simulink model "gm_sampleModel1484_1_sub_sub"  (R2023a)
settings: Solver=VariableStepAuto  StartTime=0.0  StopTime=10.0  RelTol=1e-3
libraries: hdlsllib x8, simulink x2
settings Model: Creator=user1  LastModifiedBy=user1
settings OptimizationCC: BlockReduction=off  ConditionallyExecuteInputs=off
settings DebuggingCC: InheritedTsInSrcMsg=none

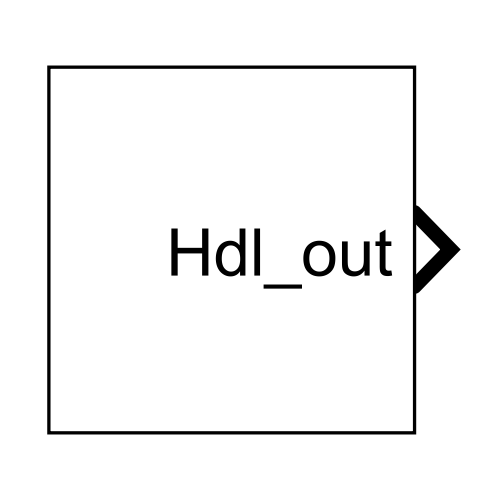
[thumbnail: Simulink's stored preview of the top-level diagram]
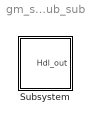
== system gm_sampleModel1484_1_sub_sub ==
  Subsystem : Subsystem

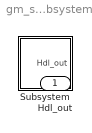
== system gm_sampleModel1484_1_sub_sub/Subsystem ==
  Subsystem : Subsystem
  Hdl_out : Outport  OutDataTypeStr=uint8

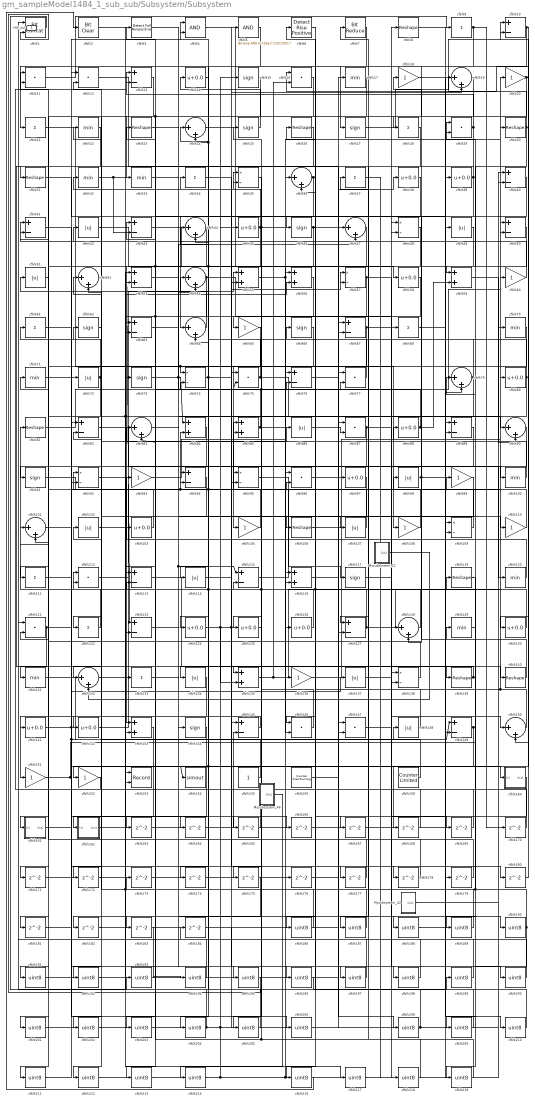
== system gm_sampleModel1484_1_sub_sub/Subsystem/Subsystem ==
  Mysubsystem_22 : Subsystem  TreatAsAtomicUnit=on  RTWFcnName=Mysubsystem_22
      settings: RTWFcnNameOpts=User specified  RTWFileNameOpts=Use function name
  Mysubsystem_42 : Subsystem  TreatAsAtomicUnit=on  RTWFcnName=Mysubsystem_42
      settings: RTWFcnNameOpts=User specified  RTWFileNameOpts=Use function name
  Mysubsystem_46 : Subsystem  TreatAsAtomicUnit=on  RTWFcnName=Mysubsystem_46
      settings: RTWFcnNameOpts=User specified  RTWFileNameOpts=Use function name
  cfblk1 : hdlsllib/Logic and Bit Operations/Bit Concat  numInputs=2
  cfblk{10,13,40..41,43,50,63,67,76,82,89,94,113,115,123,127,145,149} (18 alike) : Sum  Inputs=+-  OutDataTypeStr=uint8
  cfblk{17,22,32..33,70..71,100,120,129,131} (10 alike) : MinMax  OutDataTypeStr=uint8
  cfblk{19,24,36,44,47,52,54,64,79,83,90,101,128,132,150} (15 alike) : Sum  Inputs=|++  OutDataTypeStr=uint8
  cfblk{42,49,51,72,86,98,102,107,114,134,137,148} (12 alike) : Abs  OutDataTypeStr=uint8  SaturateOnIntegerOverflow=off
  cfblk{14,38..39,45,58,80,88,97,103,124..126,130,141..142} (15 alike) : Bias  Bias=0.0  SaturateOnIntegerOverflow=off
  cfblk{18,20,60,65,93,99,105,108,110,136,151..152} (12 alike) : Gain  OutDataTypeStr=uint8
  cfblk{8,23,26,30..31,81,106,119,139..140} (10 alike) : Reshape
  cfblk{35,48,57,74,92,95,109,138} (8 alike) : Product  Inputs=*/  OutDataTypeStr=uint8  RndMeth=Zero  SaturateOnIntegerOverflow=on
  cfblk{11..12,16,29,75,77,87,96,112,121,146..147} (12 alike) : DotProduct  OutDataTypeStr=uint8
  cfblk{9,21,28,34,37,61,68,111,122,133} (10 alike) : Sum  Inputs=+  OutDataTypeStr=uint8
  cfblk{53,55..56,59,84..85,116,135,143} (9 alike) : Sum  OutDataTypeStr=uint8
  cfblk{15,25,27,46,62,66,73,91,117,144} (10 alike) : Signum
  cfblk153 : Record  FileSettingsInternal="{\"entries\":[{\"content\":{\"excelSettings\":{\"content\":{},\"type\":\"Streamout.ExcelSettings\"}},\"type\":\"Streamout.FileSettingStorage\",\"uuid\":\"\"}],\"packageUris\":[\"http:\\/\\/schema.mathworks.com\\/mf0\\/streamout_blocks\\/R2020a\"],\"version\":\"1.0\"}"  Layout=[1 1]  SignalsInternal="{\"entries\":[{\"content\":{\"signals\":[{\"content\":{\"blockPath\":[],\"dimensions\":[1],\"domain\":\"\",\"lineColor\":\"#a2142f\",\"plots\":[1],\"port\":1,\"signalID\":17006,\"signalName\":\"cfblk204\"},\"type\":\"RecordBlkView.Signal\",\"uuid\":\"\"},{\"content\":{\"blockPath\":[],\"dimensions\":[1],\"domain\":\"\",\"lineColor\":\"#139fff\",\"plots\":[1],\"port\":2,\"signalID\":17009,\"signalName\":\"cfblk20\"},\"type\":\"RecordBlkView.Signal\",\"uuid\":\"\"}]},\"type\":\"RecordBlkView.InputSignals\",\"uuid\":\"\"}],\"packageUris\":[\"http:\\/\\/schema.mathworks.com\\/mf0\\/streamout_blocks\\/R2020a\"],\"version\":\"1.0\"}"  VisualizationBindings="{\"xyplotplugin\":{\"info\":[{\"series\":[{\"bindingParametersList\":[{\"parameter\":\"X-Axis\",\"signalID\":17006,\"signalName\":\"cfblk204\"},{\"parameter\":\"Y-Axis\",\"signalID\":17009,\"signalName\":\"cfblk20\"}],\"seriesID\":45599}],\"subplotID\":1}]}}"  CompatibilityTag=XY  st=-1
  cfblk154 : ToWorkspace  VariableName=simout  SaveFormat=Timeseries  SampleTime=-1
  cfblk155 : Constant  OutDataTypeStr=uint8  SampleTime=-1
  cfblk156 : hdlsllib/Sources/Counter Free-Running  NumBits=16  tsamp=-1
  cfblk158 : hdlsllib/Sources/Counter Limited  uplimit=7  tsamp=-1
  cfblk160 : Subsystem
      settings: LibrarySourceBlock=|
      | hdlsllib/Ports &
      | Subsystems/Subsystem
  cfblk161 : Subsystem
      settings: LibrarySourceBlock=|
      | hdlsllib/Ports &
      | Subsystems/Subsystem
  cfblk162 : Subsystem
      settings: LibrarySourceBlock=|
      | hdlsllib/Ports &
      | Subsystems/Subsystem
  cfblk{163..184} (22 alike) : Delay  SampleTime=1
  cfblk{186..206,208..214,216..219} (32 alike) : DataTypeConversion  OutDataTypeStr=uint8  SaturateOnIntegerOverflow=off  RndMeth=Floor
  cfblk2 : simulink/Logic and Bit Operations/Bit Clear  iBit=0
      settings: LibrarySourceBlock=|
      | hdlsllib/Logic and Bit
      | Operations/Bit Clear
  cfblk3 : hdlsllib/Logic and Bit Operations/Detect Fall Nonpositive  vinit=0  OutDataTypeStr=uint8
  cfblk4 : Logic  AllPortsSameDT=off  OutDataTypeStr=boolean
  cfblk5 : simulink/Logic and Bit Operations/Bitwise Operator  logicop=AND  UseBitMask=on  BitMask=bin2dec('11011001')  BitMaskRealWorld=Stored Integer
      settings: LibrarySourceBlock=|
      | hdlsllib/Logic and Bit
      | Operations/Bitwise
      | Operator
  cfblk6 : hdlsllib/Logic and Bit Operations/Detect Rise Positive  vinit=0  OutDataTypeStr=uint8
  cfblk7 : hdlsllib/Logic and Bit Operations/Bit Reduce  mode=AND
  Hdl_out : Outport  OutDataTypeStr=uint8
  wires:
  cfblk122/1 -> cfblk81/1
  cfblk113/1 -> cfblk139/1
  cfblk150/1 -> cfblk26/1, cfblk20/1
  cfblk142/1 -> cfblk55/1
  cfblk131/1 -> cfblk148/1
  cfblk4/1 -> cfblk105/1
  cfblk38/1 -> cfblk64/1
  cfblk103/1 -> cfblk92/1
  cfblk34/1 -> cfblk145/1
  cfblk19/1 -> cfblk203/1, cfblk202/1
  cfblk11/1 -> cfblk9/1
  cfblk5/1 -> cfblk204/1
  cfblk66/1 -> cfblk181/1, cfblk74/1
  cfblk22/1 -> cfblk143/1
  cfblk56/1 -> cfblk65/1
  cfblk21/1 -> cfblk108/1
  cfblk136/1 -> cfblk50/1
  cfblk18/1 -> cfblk152/1
  cfblk116/1 -> cfblk190/1
  cfblk35/1 -> cfblk125/1
  cfblk151/1 -> cfblk94/2, cfblk129/1
  cfblk95/1 -> cfblk117/1
  cfblk46/1 -> cfblk38/1, cfblk133/1
  cfblk42/1 -> cfblk58/1
  cfblk36/1 -> cfblk63/1, cfblk146/1
  cfblk64/1 -> cfblk51/1
  cfblk132/1 -> cfblk86/1
  cfblk29/1 -> cfblk187/1, cfblk13/2
  cfblk152/1 -> cfblk13/1
  cfblk98/1 -> cfblk210/1, cfblk18/1
  cfblk115/1 -> cfblk50/2
  cfblk25/1 -> cfblk14/1
  cfblk13/1 -> cfblk142/1
  cfblk9/1 -> cfblk170/1, cfblk28/1
  cfblk76/1 -> cfblk208/1
  cfblk109/1 -> cfblk85/1
  cfblk100/1 -> cfblk62/1
  cfblk87/1 -> cfblk191/1, cfblk149/2
  cfblk47/1 -> cfblk124/1, cfblk123/1
  cfblk135/1 -> cfblk16/2, cfblk80/1
  cfblk74/1 -> cfblk19/2, cfblk4/1
  cfblk127/1 -> cfblk41/2, cfblk119/1
  cfblk81/1 -> cfblk60/1
  cfblk73/1 -> cfblk47/2, cfblk84/1
  cfblk16/1 -> cfblk33/1
  cfblk50/1 -> cfblk146/2
  cfblk80/1 -> cfblk35/2, cfblk161/1(In1), cfblk123/2
  cfblk86/1 -> cfblk87/2
  cfblk155/1 -> cfblk54/1
  cfblk105/1 -> cfblk83/1, cfblk84/2
  cfblk30/1 -> cfblk59/1, cfblk16/1
  cfblk15/1 -> cfblk73/1
  cfblk134/1 -> cfblk151/1
  cfblk43/1 -> cfblk136/1
  cfblk112/1 -> cfblk54/2
  cfblk110/1 -> cfblk61/1
  cfblk51/1 -> cfblk111/1
  cfblk138/1 -> cfblk71/1
  cfblk90/1 -> cfblk127/1
  cfblk77/1 -> cfblk32/1
  cfblk102/1 -> cfblk85/2
  cfblk65/1 -> cfblk122/1
  cfblk31/1 -> cfblk46/1
  cfblk106/1 -> cfblk88/1
  cfblk75/1 -> cfblk89/2, cfblk34/1
  cfblk10/1 -> cfblk150/2, cfblk21/1
  cfblk27/1 -> cfblk10/1
  cfblk125/1 -> cfblk95/1
  cfblk93/1 -> cfblk56/1
  cfblk20/1 -> cfblk153/2, cfblk130/1
  cfblk67/1 -> cfblk127/2, cfblk68/1
  cfblk84/1 -> cfblk91/1
  cfblk53/1 -> cfblk106/1
  cfblk6/1 -> cfblk186/1
  cfblk107/1 -> cfblk43/1, cfblk74/2
  cfblk32/1 -> cfblk43/2, cfblk140/1
  cfblk62/1 -> cfblk162/1(In1)
  cfblk128/1 -> cfblk112/1
  cfblk7/1 -> cfblk27/1
  cfblk117/1 -> cfblk8/1
  cfblk33/1 -> cfblk90/1
  cfblk57/1 -> cfblk213/1, cfblk100/1
  cfblk12/1 -> cfblk97/1
  cfblk139/1 -> cfblk134/1, cfblk29/1
  cfblk63/1 -> cfblk110/1
  cfblk141/1 -> cfblk165/1, cfblk82/1
  cfblk24/1 -> cfblk109/1
  cfblk149/1 -> cfblk168/1, cfblk99/1
  cfblk45/1 -> cfblk63/2, cfblk12/2, cfblk175/1, cfblk36/1
  cfblk71/1 -> cfblk160/1(In1)
  cfblk121/1 -> cfblk4/2, cfblk131/1
  cfblk146/1 -> cfblk25/1
  cfblk61/1 -> cfblk12/1
  cfblk108/1 -> cfblk24/2, cfblk24/1
  cfblk120/1 -> cfblk93/1
  cfblk59/1 -> cfblk90/2
  cfblk23/1 -> cfblk115/1, cfblk144/1
  cfblk49/1 -> cfblk114/1
  cfblk70/1 -> cfblk132/1
  cfblk89/1 -> cfblk135/1
  cfblk156/1 -> cfblk47/1
  cfblk91/1 -> cfblk98/1
  cfblk37/1 -> cfblk218/1
  cfblk92/1 -> cfblk56/2
  cfblk79/1 -> cfblk107/1, cfblk36/2
  cfblk158/1 -> cfblk82/2
  cfblk60/1 -> cfblk41/1
  cfblk126/1 -> cfblk11/2, cfblk75/2, cfblk35/1
  cfblk130/1 -> cfblk66/1, cfblk94/1, cfblk52/2
  cfblk82/1 -> cfblk120/1
  cfblk145/1 -> cfblk141/1
  cfblk72/1 -> cfblk92/2, cfblk11/1
  cfblk140/1 -> cfblk42/1
  cfblk14/1 -> cfblk174/1, cfblk154/1
  cfblk54/1 -> cfblk138/1, cfblk83/2, cfblk143/2
  cfblk124/1 -> cfblk135/2, cfblk57/2, cfblk138/2
  cfblk44/1 -> cfblk163/1, cfblk101/2
  cfblk58/1 -> cfblk113/1
  cfblk161/1(Out1) -> cfblk137/1, cfblk149/1
  cfblk55/1 -> cfblk67/2, cfblk30/1
  cfblk162/1(Out1) -> cfblk128/1
  cfblk88/1 -> cfblk59/2, cfblk44/2
  cfblk39/1 -> cfblk31/1, cfblk128/2
  cfblk68/1 -> cfblk19/1
  cfblk148/1 -> cfblk7/1
  cfblk97/1 -> cfblk103/1
  cfblk8/1 -> cfblk150/1
  cfblk85/1 -> cfblk23/1, cfblk57/1
  cfblk52/1 -> cfblk22/1
  cfblk163/1 -> cfblk29/2
  cfblk41/1 -> cfblk164/1
  cfblk164/1 -> cfblk145/2
  cfblk165/1 -> cfblk113/2
  cfblk123/1 -> cfblk166/1
  cfblk166/1 -> cfblk89/1
  cfblk99/1 -> cfblk167/1
  cfblk167/1 -> cfblk109/2
  cfblk168/1 -> cfblk112/2
  cfblk137/1 -> cfblk169/1
  cfblk169/1 -> cfblk101/1
  cfblk170/1 -> cfblk52/1
  cfblk28/1 -> cfblk171/1
  cfblk171/1 -> cfblk95/2
  cfblk94/1 -> cfblk172/1
  cfblk172/1 -> cfblk53/2
  cfblk173/1 -> cfblk147/1
  cfblk174/1 -> cfblk55/2
  cfblk176/1 -> cfblk67/1
  cfblk114/1 -> cfblk177/1
  cfblk177/1 -> cfblk77/1
  cfblk111/1 -> cfblk178/1
  cfblk178/1 -> cfblk44/1
  cfblk179/1 -> cfblk121/2
  cfblk83/1 -> cfblk180/1
  cfblk180/1 -> cfblk10/2
  cfblk26/1 -> cfblk182/1
  cfblk182/1 -> cfblk87/1
  cfblk144/1 -> cfblk183/1
  cfblk186/1 -> cfblk53/1, cfblk102/1
  cfblk187/1 -> cfblk6/1
  cfblk3/1 -> cfblk188/1
  cfblk188/1 -> cfblk39/1
  cfblk129/1 -> cfblk189/1
  cfblk189/1 -> cfblk3/1
  cfblk190/1 -> cfblk209/1, cfblk75/1, cfblk79/1
  cfblk191/1 -> cfblk116/1
  cfblk175/1 -> cfblk192/1
  cfblk192/1 -> cfblk116/2
  cfblk1/1 -> cfblk193/1
  cfblk193/1 -> cfblk147/2
  cfblk183/1 -> cfblk194/1
  cfblk194/1 -> cfblk1/1
  cfblk181/1 -> cfblk195/1
  cfblk195/1 -> cfblk1/2
  cfblk184/1 -> cfblk196/1
  cfblk133/1 -> cfblk197/1
  cfblk197/1 -> cfblk184/1
  cfblk96/1 -> cfblk198/1
  cfblk198/1 -> cfblk77/2
  cfblk196/1 -> cfblk199/1
  cfblk199/1 -> cfblk96/1
  cfblk147/1 -> cfblk200/1
  cfblk200/1 -> cfblk96/2
  cfblk17/1 -> cfblk201/1
  cfblk201/1 -> cfblk49/1
  cfblk202/1 -> cfblk17/1
  cfblk203/1 -> cfblk5/1
  cfblk204/1 -> cfblk153/1, cfblk45/1, cfblk176/1
  cfblk40/1 -> cfblk205/1
  cfblk205/1 -> cfblk121/1
  cfblk101/1 -> cfblk206/1
  cfblk206/1 -> cfblk40/1
  cfblk208/1 -> cfblk64/2, cfblk179/1
  cfblk209/1 -> cfblk76/1
  cfblk210/1 -> cfblk76/2
  cfblk48/1 -> cfblk211/1
  cfblk211/1 -> cfblk72/1
  cfblk143/1 -> cfblk212/1
  cfblk212/1 -> cfblk48/1
  cfblk213/1 -> cfblk48/2
  cfblk214/1 -> cfblk15/1, cfblk126/1, cfblk79/2
  cfblk160/1(Out1) -> cfblk216/1
  cfblk216/1 -> cfblk2/1
  cfblk2/1 -> cfblk217/1
  cfblk217/1 -> cfblk70/1
  cfblk218/1 -> cfblk115/2, cfblk173/1
  cfblk119/1 -> cfblk219/1
  cfblk219/1 -> cfblk37/1
  Mysubsystem_22/1(Out1) -> cfblk132/2
  Mysubsystem_42/1(Out1) -> cfblk40/2
  Mysubsystem_46/1(Out1) -> cfblk214/1

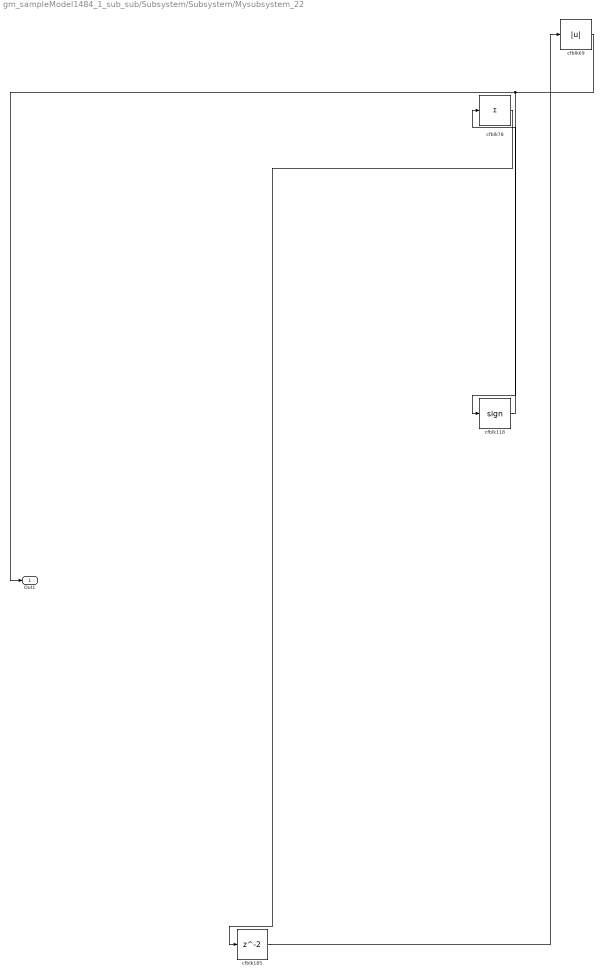
== system gm_sampleModel1484_1_sub_sub/Subsystem/Subsystem/Mysubsystem_22 ==
  cfblk118 : Signum
  cfblk185 : Delay  SampleTime=1
  cfblk69 : Abs  SaturateOnIntegerOverflow=off
  cfblk78 : Sum  Inputs=+
  Out1 : Outport
  wires:
  cfblk78/1 -> cfblk185/1
  cfblk69/1 -> cfblk118/1, Out1/1
  cfblk185/1 -> cfblk69/1
  cfblk118/1 -> cfblk78/1

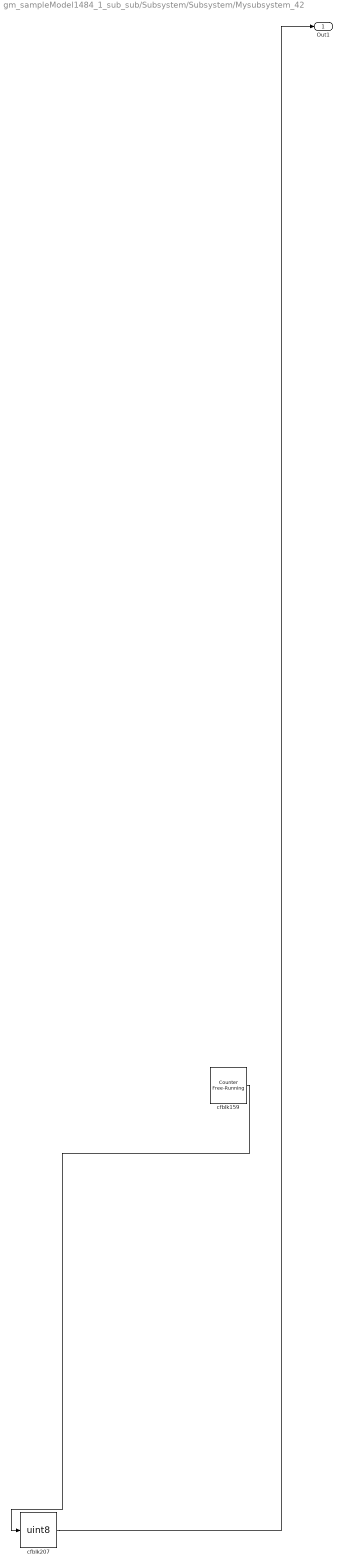
== system gm_sampleModel1484_1_sub_sub/Subsystem/Subsystem/Mysubsystem_42 ==
  cfblk159 : hdlsllib/Sources/Counter Free-Running  NumBits=16  tsamp=-1
  cfblk207 : DataTypeConversion  OutDataTypeStr=uint8  SaturateOnIntegerOverflow=off  RndMeth=Floor
  Out1 : Outport
  wires:
  cfblk207/1 -> Out1/1
  cfblk159/1 -> cfblk207/1

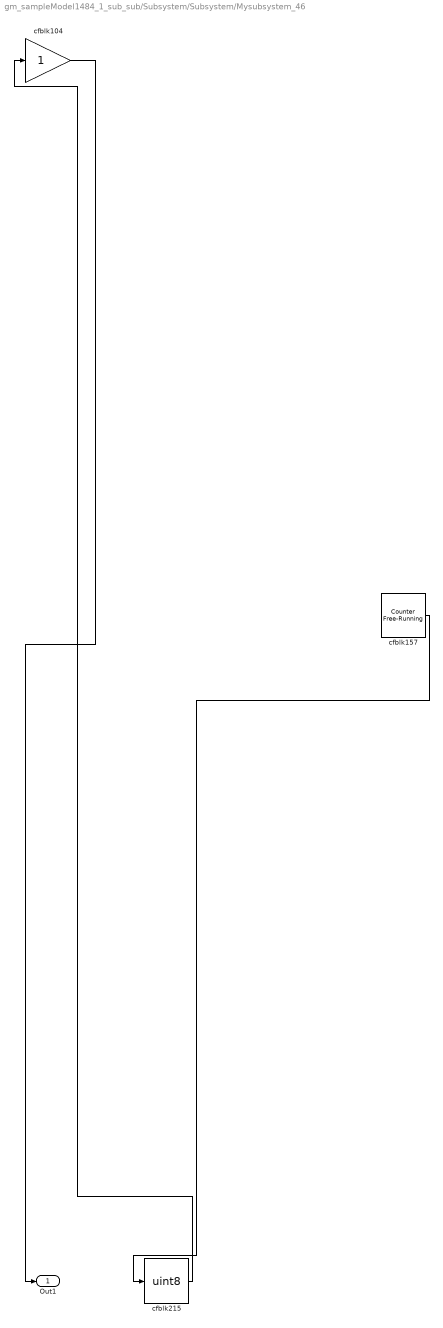
== system gm_sampleModel1484_1_sub_sub/Subsystem/Subsystem/Mysubsystem_46 ==
  cfblk104 : Gain
  cfblk157 : hdlsllib/Sources/Counter Free-Running  NumBits=16  tsamp=-1
  cfblk215 : DataTypeConversion  OutDataTypeStr=uint8  SaturateOnIntegerOverflow=off  RndMeth=Floor
  Out1 : Outport
  wires:
  cfblk215/1 -> cfblk104/1
  cfblk157/1 -> cfblk215/1
  cfblk104/1 -> Out1/1

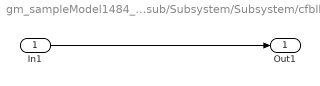
== system gm_sampleModel1484_1_sub_sub/Subsystem/Subsystem/cfblk160 ==
  In1 : Inport
  Out1 : Outport
  wires:
  In1/1 -> Out1/1

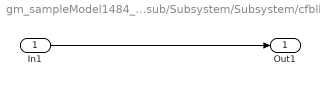
== system gm_sampleModel1484_1_sub_sub/Subsystem/Subsystem/cfblk161 ==
  In1 : Inport
  Out1 : Outport
  wires:
  In1/1 -> Out1/1

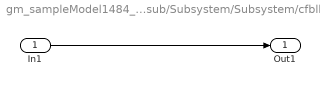
== system gm_sampleModel1484_1_sub_sub/Subsystem/Subsystem/cfblk162 ==
  In1 : Inport
  Out1 : Outport
  wires:
  In1/1 -> Out1/1
